simulink model "loopgain_stability_nyquist"  (Simulink 8.1)
settings: Solver=ode45  StartTime=0.0  StopTime=10.0  RelTol=1e-3
undefined symbols (not defined in the file or in its folder): fb, Kp, plant
settings Model: Creator=mainster  LastModifiedBy=mainster
settings DataIOCC: SignalLoggingSaveFormat=Dataset
settings OptimizationCC: ExpressionDepthLimit=128
settings DebuggingCC: SolverPrmCheckMsg=none  FcnCallInpInsideContextMsg=EnableAllAsError
settings GRTTargetCC: CombineOutputUpdateFcns=on  GRTInterface=off

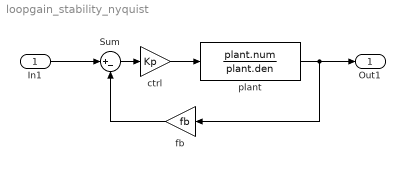
== system loopgain_stability_nyquist ==
  In1 : Inport
  Sum : Sum  Inputs=|+-
  ctrl : Gain  Gain=Kp
  fb : Gain  Gain=fb
  plant : TransferFcn  Numerator=plant.num  Denominator=plant.den
  Out1 : Outport
  wires:
  ctrl/1 -> plant/1
  plant/1 -> fb/1, Out1/1
  In1/1 -> Sum/1
  fb/1 -> Sum/2
  Sum/1 -> ctrl/1
